simulink model "quartersuspensiontire"  (R2020b)
settings: Solver=VariableStepAuto  StartTime=0.0  StopTime=5  RelTol=1e-3
values from neighbouring files (symbols this model uses):
  K = lqr(A,B,Q_pd,rho_pd)    [accel_jerk_ctrl_testbed.m]    (also in quartersuspensionscript.m)
undefined symbols (not defined in the file or in its folder): b_damper, k_spring, k_wheel, m_car, m_wheel
settings Model: Creator=anishabhangui  LastModifiedBy=anishabhangui
settings DebuggingCC: UnderSpecifiedDimensionMsg=warning

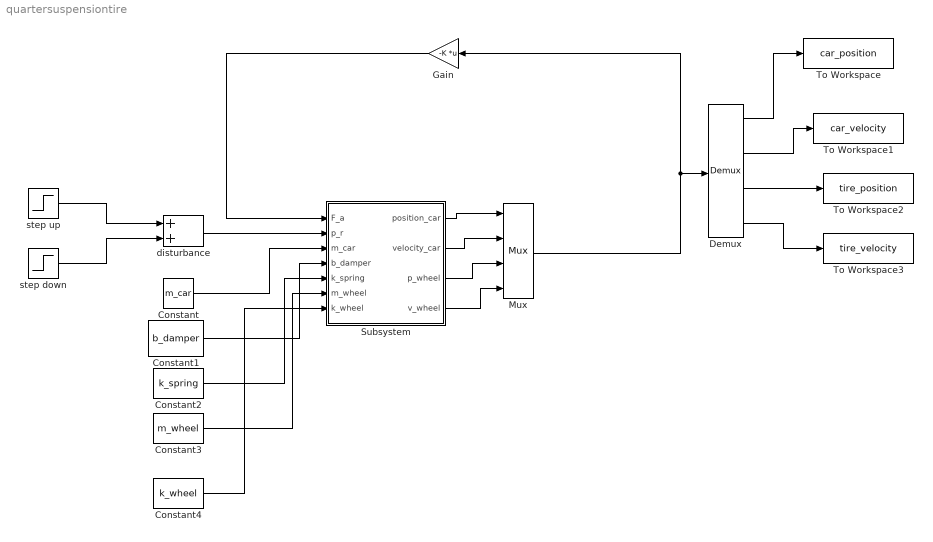
== system quartersuspensiontire ==
  Constant : Constant  Value=m_car
  Constant1 : Constant  Value=b_damper
  Constant2 : Constant  Value=k_spring
  Constant3 : Constant  Value=m_wheel
  Constant4 : Constant  Value=k_wheel
  Demux : Demux
  Gain : Gain  Gain=-K  Multiplication=Matrix(K*u)
  Mux : Mux
  Subsystem : Subsystem
  To Workspace : ToWorkspace  VariableName=car_position  SaveFormat=Timeseries  SampleTime=-1
  To Workspace1 : ToWorkspace  VariableName=car_velocity  SaveFormat=Timeseries  SampleTime=-1
  To Workspace2 : ToWorkspace  VariableName=tire_position  SaveFormat=Timeseries  SampleTime=-1
  To Workspace3 : ToWorkspace  VariableName=tire_velocity  SaveFormat=Timeseries  SampleTime=-1
  disturbance : Sum
  step down : Step  After=-1  SampleTime=0
  step up : Step  Time=0  SampleTime=0
  wires:
  step up/1 -> disturbance/1
  disturbance/1 -> Subsystem/2(p_r)
  step down/1 -> disturbance/2
  Constant/1 -> Subsystem/3(m_car)
  Constant1/1 -> Subsystem/4(b_damper)
  Constant2/1 -> Subsystem/5(k_spring)
  Constant3/1 -> Subsystem/6(m_wheel)
  Constant4/1 -> Subsystem/7(k_wheel)
  Subsystem/1(position_car) -> Mux/1
  Subsystem/2(velocity_car) -> Mux/2
  Subsystem/3(p_wheel) -> Mux/3
  Subsystem/4(v_wheel) -> Mux/4
  Mux/1 -> Gain/1, Demux/1
  Gain/1 -> Subsystem/1(F_a)
  Demux/1 -> To Workspace/1
  Demux/2 -> To Workspace1/1
  Demux/3 -> To Workspace2/1
  Demux/4 -> To Workspace3/1

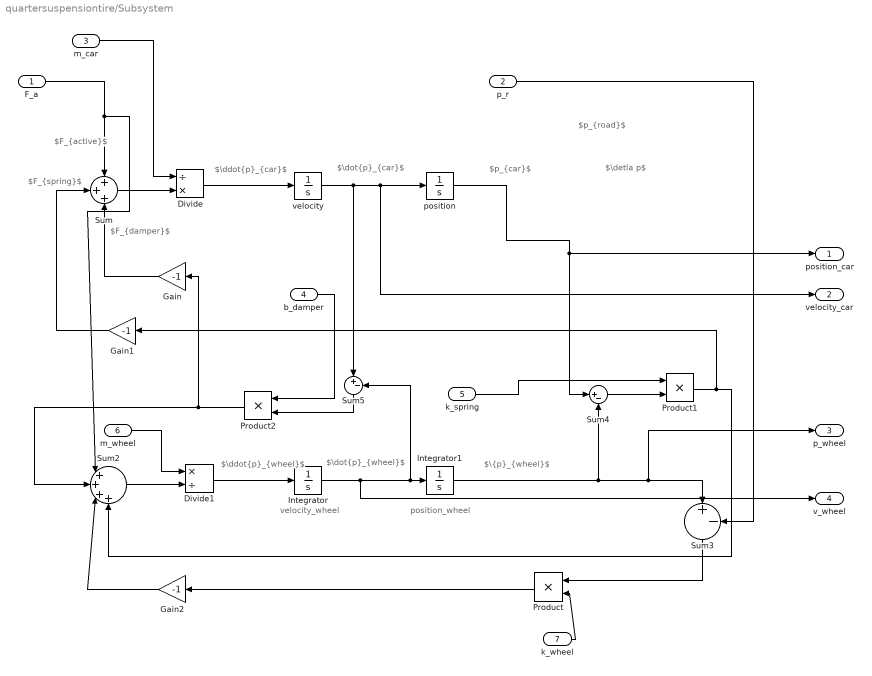
== system quartersuspensiontire/Subsystem ==
  note: $\dot{p}_{wheel}$
  note: position_wheel
  note: velocity_wheel
  note: $\ddot{p}_{wheel}$
  note: $\ddot{p}_{car}$
  note: $\detla p$
  note: $\dot{p}_{car}$
  note: $F_{active}$
  note: $p_{car}$
  note: $p_{road}$
  note: $F_{damper}$
  note: $F_{spring}$
  note: $\{p}_{wheel}$
  F_a : Inport
  p_r : Inport  Port=2
  m_car : Inport  Port=3
  b_damper : Inport  Port=4
  k_spring : Inport  Port=5
  m_wheel : Inport  Port=6
  k_wheel : Inport  Port=7
  Divide : Product  Inputs=/*
  Divide1 : Product  Inputs=*/
  Gain : Gain  Gain=-1
  Gain1 : Gain  Gain=-1
  Gain2 : Gain  Gain=-1
  Integrator : Integrator
  Integrator1 : Integrator
  Product : Product
  Product1 : Product
  Product2 : Product
  Sum : Sum  Inputs=+++
  Sum2 : Sum  Inputs=|++++
  Sum3 : Sum  Inputs=|+-
  Sum4 : Sum  Inputs=|+-
  Sum5 : Sum  Inputs=|+-
  position : Integrator
  velocity : Integrator
  position_car : Outport
  velocity_car : Outport  Port=2
  p_wheel : Outport  Port=3
  v_wheel : Outport  Port=4
  wires:
  Gain1/1 -> Sum/2
  k_wheel/1 -> Product/2
  Gain/1 -> Sum/3
  Product/1 -> Gain2/1
  m_wheel/1 -> Divide1/1
  Divide1/1 -> Integrator/1
  Integrator1/1 -> Sum4/2, p_wheel/1, Sum3/1
  k_spring/1 -> Product1/1
  Divide/1 -> velocity/1
  Sum4/1 -> Product1/2
  Sum3/1 -> Product/1
  Gain2/1 -> Sum2/3
  Product1/1 -> Gain1/1, Sum2/4
  Sum2/1 -> Divide1/2
  Sum5/1 -> Product2/2
  position/1 -> position_car/1, Sum4/1
  Sum/1 -> Divide/2
  b_damper/1 -> Product2/1
  Product2/1 -> Gain/1, Sum2/2
  m_car/1 -> Divide/1
  F_a/1 -> Sum2/1, Sum/1
  velocity/1 -> Sum5/1, velocity_car/1, position/1
  Integrator/1 -> v_wheel/1, Sum5/2, Integrator1/1
  p_r/1 -> Sum3/2
